simulink subsystem "springLinear_mdl"  (R2023a)
settings: Solver=VariableStepAuto  StartTime=0.0  StopTime=10.0  RelTol=1e-3
model mask{obj=obj}
  mask prompts: obj "Spring Object:"
settings Model: Creator=grouleau  LastModifiedBy=grouleau

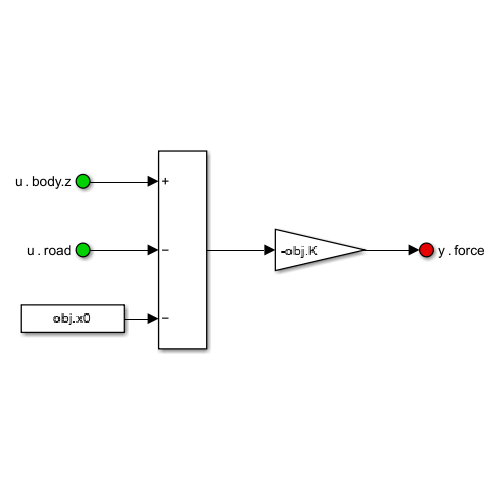
[thumbnail: Simulink's stored preview of the top-level diagram]
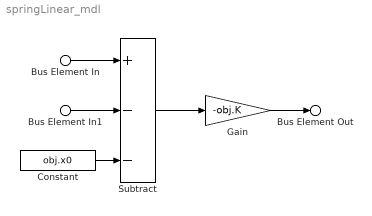
== system springLinear_mdl ==
  Bus Element In : Inport  PortName=u  Element=body.z
  Bus Element In1 : Inport  PortName=u  Element=road
  Constant : Constant  Value=obj.x0
  Gain : Gain  Gain=-obj.K
  Subtract : Sum  Inputs=+--
  Bus Element Out : Outport  PortName=y  Element=force
  wires:
  Bus Element In1/1 -> Subtract/2
  Subtract/1 -> Gain/1
  Bus Element In/1 -> Subtract/1
  Constant/1 -> Subtract/3
  Gain/1 -> Bus Element Out/1
